simulink model "RL_EKF_"  (R2019b)
settings: Solver=VariableStepAuto  StartTime=0.0  StopTime=10.0  RelTol=1e-3
PreLoadFcn:
  | modelDir = fileparts(get_param(bdroot, 'FileName'));
  | addpath(fullfile(modelDir,'../../Parameters'));
  | addpath(fullfile(modelDir,'../../Estimation/RL-EKF'));
  | 
  | Parameters_Model
  | Parameters_Simulation
  | Parameters_Estimators
InitFcn:
  | Parameters_Model
  | Parameters_Simulation
  | Parameters_Estimators
undefined symbols (not defined in the file): Ke, RLekf_P_init, RLekf_X_init
settings Model: Creator=Thomas  LastModifiedBy=thomas.jespersen
settings DataIOCC: ReturnWorkspaceOutputs=off
settings DebuggingCC: ArithmeticOperatorsInVariantConditions=warning
settings SFSimCC: SimUseLocalCustomCode=off  CustomCodeUndefinedFunction=UseInterfaceOnly
settings RTWCC: RTWUseLocalCustomCode=off

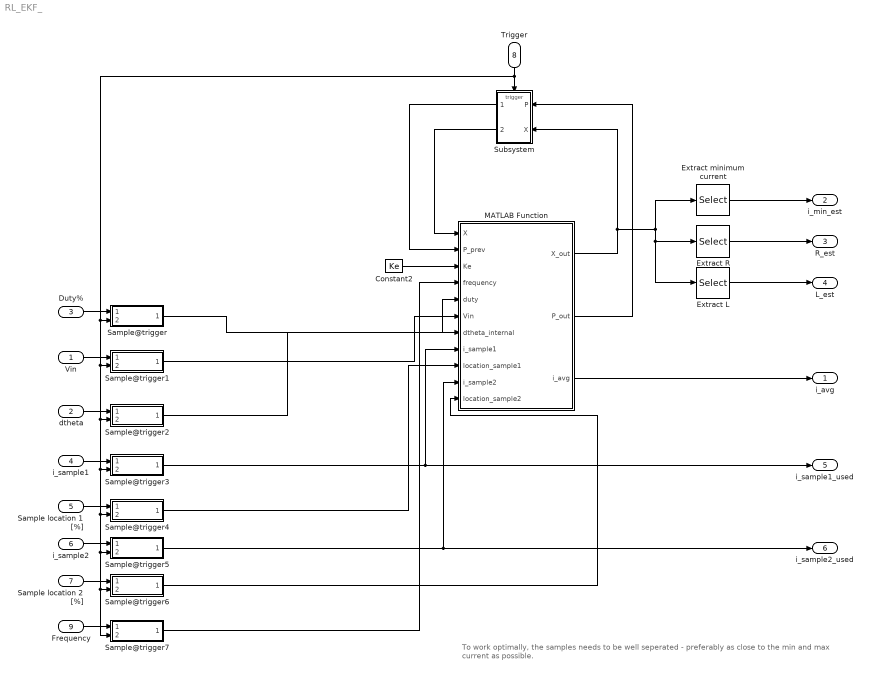
== system RL_EKF_ ==
  note: To work optimally, the samples needs to be well seperated - preferably as close to the min and max current as possible.
  Vin : Inport  OutDataTypeStr=double
  dtheta : Inport  Port=2  OutDataTypeStr=double
  Duty% : Inport  Port=3  OutDataTypeStr=double
  i_sample1 : Inport  Port=4  OutDataTypeStr=double
  Sample location 1 [%] : Inport  Port=5  OutDataTypeStr=double
  i_sample2 : Inport  Port=6  OutDataTypeStr=double
  Sample location 2 [%] : Inport  Port=7  OutDataTypeStr=double
  Trigger : Inport  Port=8  OutDataTypeStr=boolean
  Frequency : Inport  Port=9  OutDataTypeStr=double
  Constant2 : Constant  Value=Ke
  Extract L : Selector  InputPortWidth=3  IndexOptions=Index vector (dialog)  Indices=[3]  OutputSizes=1
  Extract R : Selector  InputPortWidth=3  IndexOptions=Index vector (dialog)  Indices=[2]  OutputSizes=1
  Extract minimum current : Selector  InputPortWidth=3  IndexOptions=Index vector (dialog)  Indices=[1]  OutputSizes=1
  MATLAB Function : MATLAB Function  TreatAsAtomicUnit=on
  Sample@trigger : Subsystem
  Sample@trigger1 : Subsystem
  Sample@trigger2 : Subsystem
  Sample@trigger3 : Subsystem
  Sample@trigger4 : Subsystem
  Sample@trigger5 : Subsystem
  Sample@trigger6 : Subsystem
  Sample@trigger7 : Subsystem
  Subsystem : Subsystem
  i_avg : Outport  VectorParamsAs1DForOutWhenUnconnected=off
  i_min_est : Outport  Port=2  VectorParamsAs1DForOutWhenUnconnected=off
  R_est : Outport  Port=3  VectorParamsAs1DForOutWhenUnconnected=off
  L_est : Outport  Port=4  VectorParamsAs1DForOutWhenUnconnected=off
  i_sample1_used : Outport  Port=5  VectorParamsAs1DForOutWhenUnconnected=off
  i_sample2_used : Outport  Port=6  VectorParamsAs1DForOutWhenUnconnected=off
  wires:
  Constant2/1 -> MATLAB Function/3(Ke)
  Sample@trigger2/1(Sample) -> MATLAB Function/7(dtheta_internal)
  Sample@trigger7/1(Sample) -> MATLAB Function/4(frequency)
  Sample@trigger3/1(Sample) -> i_sample1_used/1, MATLAB Function/8(i_sample1)
  Sample@trigger5/1(Sample) -> i_sample2_used/1, MATLAB Function/10(i_sample2)
  MATLAB Function/3(i_avg) -> i_avg/1
  Extract minimum current/1 -> i_min_est/1
  Extract R/1 -> R_est/1
  Extract L/1 -> L_est/1
  Sample@trigger4/1(Sample) -> MATLAB Function/9(location_sample1)
  Sample@trigger6/1(Sample) -> MATLAB Function/11(location_sample2)
  MATLAB Function/1(X_out) -> Subsystem/2(X), Extract minimum current/1, Extract L/1, Extract R/1
  Trigger/1 -> Sample@trigger1/2(Trigger), Sample@trigger2/2(Trigger), Sample@trigger3/2(Trigger), Sample@trigger4/2(Trigger), Sample@trigger7/2(Trigger), Sample@trigger6/2(Trigger), Sample@trigger5/2(Trigger), Sample@trigger/2(Trigger), Subsystem/Trigger
  MATLAB Function/2(P_out) -> Subsystem/1(P)
  Subsystem/2(X_prev) -> MATLAB Function/1(X)
  Subsystem/1(P_prev) -> MATLAB Function/2(P_prev)
  Duty%/1 -> Sample@trigger/1(Signal)
  Vin/1 -> Sample@trigger1/1(Signal)
  dtheta/1 -> Sample@trigger2/1(Signal)
  Sample@trigger1/1(Sample) -> MATLAB Function/6(Vin)
  Sample@trigger/1(Sample) -> MATLAB Function/5(duty)
  i_sample1/1 -> Sample@trigger3/1(Signal)
  Sample location 1 [%]/1 -> Sample@trigger4/1(Signal)
  i_sample2/1 -> Sample@trigger5/1(Signal)
  Sample location 2 [%]/1 -> Sample@trigger6/1(Signal)
  Frequency/1 -> Sample@trigger7/1(Signal)

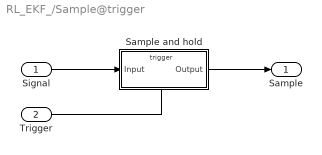
== system RL_EKF_/Sample@trigger ==
  Signal : Inport
  Trigger : Inport  Port=2
  Sample and hold : Subsystem
  Sample : Outport  VectorParamsAs1DForOutWhenUnconnected=off
  wires:
  Signal/1 -> Sample and hold/1(Input)
  Sample and hold/1(Output) -> Sample/1
  Trigger/1 -> Sample and hold/Trigger

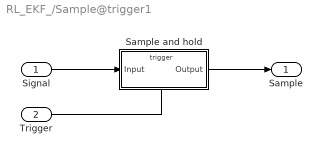
== system RL_EKF_/Sample@trigger1 ==
  Signal : Inport
  Trigger : Inport  Port=2
  Sample and hold : Subsystem
  Sample : Outport  VectorParamsAs1DForOutWhenUnconnected=off
  wires:
  Signal/1 -> Sample and hold/1(Input)
  Sample and hold/1(Output) -> Sample/1
  Trigger/1 -> Sample and hold/Trigger

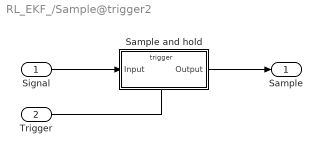
== system RL_EKF_/Sample@trigger2 ==
  Signal : Inport
  Trigger : Inport  Port=2
  Sample and hold : Subsystem
  Sample : Outport  VectorParamsAs1DForOutWhenUnconnected=off
  wires:
  Signal/1 -> Sample and hold/1(Input)
  Sample and hold/1(Output) -> Sample/1
  Trigger/1 -> Sample and hold/Trigger

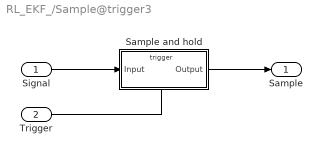
== system RL_EKF_/Sample@trigger3 ==
  Signal : Inport
  Trigger : Inport  Port=2
  Sample and hold : Subsystem
  Sample : Outport  VectorParamsAs1DForOutWhenUnconnected=off
  wires:
  Signal/1 -> Sample and hold/1(Input)
  Sample and hold/1(Output) -> Sample/1
  Trigger/1 -> Sample and hold/Trigger

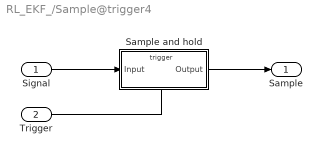
== system RL_EKF_/Sample@trigger4 ==
  Signal : Inport
  Trigger : Inport  Port=2
  Sample and hold : Subsystem
  Sample : Outport  VectorParamsAs1DForOutWhenUnconnected=off
  wires:
  Signal/1 -> Sample and hold/1(Input)
  Sample and hold/1(Output) -> Sample/1
  Trigger/1 -> Sample and hold/Trigger

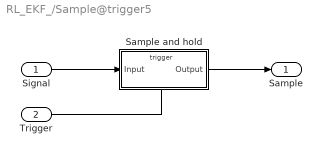
== system RL_EKF_/Sample@trigger5 ==
  Signal : Inport
  Trigger : Inport  Port=2
  Sample and hold : Subsystem
  Sample : Outport  VectorParamsAs1DForOutWhenUnconnected=off
  wires:
  Signal/1 -> Sample and hold/1(Input)
  Sample and hold/1(Output) -> Sample/1
  Trigger/1 -> Sample and hold/Trigger

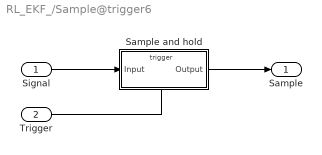
== system RL_EKF_/Sample@trigger6 ==
  Signal : Inport
  Trigger : Inport  Port=2
  Sample and hold : Subsystem
  Sample : Outport  VectorParamsAs1DForOutWhenUnconnected=off
  wires:
  Signal/1 -> Sample and hold/1(Input)
  Sample and hold/1(Output) -> Sample/1
  Trigger/1 -> Sample and hold/Trigger

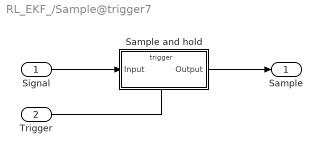
== system RL_EKF_/Sample@trigger7 ==
  Signal : Inport
  Trigger : Inport  Port=2
  Sample and hold : Subsystem
  Sample : Outport  VectorParamsAs1DForOutWhenUnconnected=off
  wires:
  Signal/1 -> Sample and hold/1(Input)
  Sample and hold/1(Output) -> Sample/1
  Trigger/1 -> Sample and hold/Trigger

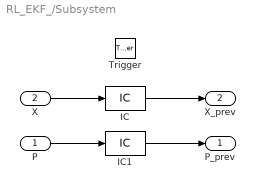
== system RL_EKF_/Subsystem ==
  P : Inport  LatchByDelayingOutsideSignal=on
  X : Inport  Port=2  LatchByDelayingOutsideSignal=on
  Trigger : TriggerPort  VariantControl=Variant  PortDimensions=1
  IC : InitialCondition  Value=RLekf_X_init
  IC1 : InitialCondition  Value=RLekf_P_init
  P_prev : Outport  VectorParamsAs1DForOutWhenUnconnected=off
  X_prev : Outport  Port=2  VectorParamsAs1DForOutWhenUnconnected=off
  wires:
  X/1 -> IC/1
  P/1 -> IC1/1
  IC/1 -> X_prev/1
  IC1/1 -> P_prev/1

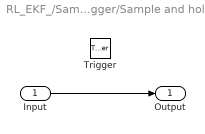
== system RL_EKF_/Sample@trigger/Sample and hold ==
  Input : Inport
  Trigger : TriggerPort  VariantControl=Variant  PortDimensions=1
  Output : Outport  VectorParamsAs1DForOutWhenUnconnected=off
  wires:
  Input/1 -> Output/1

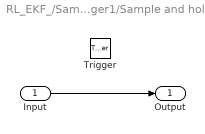
== system RL_EKF_/Sample@trigger1/Sample and hold ==
  Input : Inport
  Trigger : TriggerPort  VariantControl=Variant  PortDimensions=1
  Output : Outport  VectorParamsAs1DForOutWhenUnconnected=off
  wires:
  Input/1 -> Output/1

== system RL_EKF_/Sample@trigger2/Sample and hold ==
  Input : Inport
  Trigger : TriggerPort  VariantControl=Variant  PortDimensions=1
  Output : Outport  VectorParamsAs1DForOutWhenUnconnected=off
  wires:
  Input/1 -> Output/1

== system RL_EKF_/Sample@trigger3/Sample and hold ==
  Input : Inport
  Trigger : TriggerPort  VariantControl=Variant  PortDimensions=1
  Output : Outport  VectorParamsAs1DForOutWhenUnconnected=off
  wires:
  Input/1 -> Output/1

== system RL_EKF_/Sample@trigger4/Sample and hold ==
  Input : Inport
  Trigger : TriggerPort  VariantControl=Variant  PortDimensions=1
  Output : Outport  VectorParamsAs1DForOutWhenUnconnected=off
  wires:
  Input/1 -> Output/1

== system RL_EKF_/Sample@trigger5/Sample and hold ==
  Input : Inport
  Trigger : TriggerPort  VariantControl=Variant  PortDimensions=1
  Output : Outport  VectorParamsAs1DForOutWhenUnconnected=off
  wires:
  Input/1 -> Output/1

== system RL_EKF_/Sample@trigger6/Sample and hold ==
  Input : Inport
  Trigger : TriggerPort  VariantControl=Variant  PortDimensions=1
  Output : Outport  VectorParamsAs1DForOutWhenUnconnected=off
  wires:
  Input/1 -> Output/1

== system RL_EKF_/Sample@trigger7/Sample and hold ==
  Input : Inport
  Trigger : TriggerPort  VariantControl=Variant  PortDimensions=1
  Output : Outport  VectorParamsAs1DForOutWhenUnconnected=off
  wires:
  Input/1 -> Output/1

== matlab function RL_EKF_/MATLAB Function ==
  data: X input; X_out output; P_prev input; Ke input; frequency input; duty input; Vin input; dtheta_internal input; i_sample1 input; location_sample1 input; P_out output; i_avg output; i_sample2 input; location_sample2 input
function [X_out, P_out, i_avg] = RL_EKF_(X, P_prev, ...
    Ke, ... % constants/parameters
    frequency, duty, Vin, dtheta_internal, ... % inputs (u)
    i_sample1, location_sample1, ...
    i_sample2, location_sample2)  % measurements (z)

%     [X_out, P_out, i_avg] = RL_EKF(X, P_prev, ...
%         Ke, ... % constants/parameters
%         frequency, duty, Vin, dtheta_internal, ... % inputs (u)
%         i_sample2, i_sample1);  % measurements (z)

    [X_out, P_out, i_avg] = RL_EKF2(X, P_prev, ...
        Ke, ... % constants/parameters
        frequency, duty, Vin, dtheta_internal, ... % inputs (u)
        i_sample1, location_sample1, ...
        i_sample2, location_sample2);  % measurements (z)

end
